simulink subsystem "PID_controller_subsys"  (R2022b)
settings: Solver=VariableStepAuto  StartTime=0.0  StopTime=10.0  RelTol=1e-3
settings Model: Creator=seobokyeong  LastModifiedBy=kevin

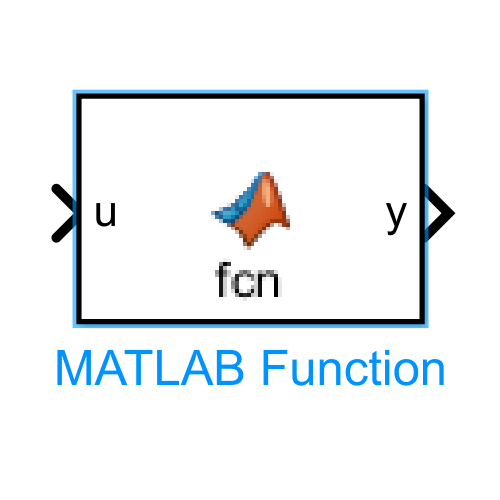
[thumbnail: Simulink's stored preview of the top-level diagram]
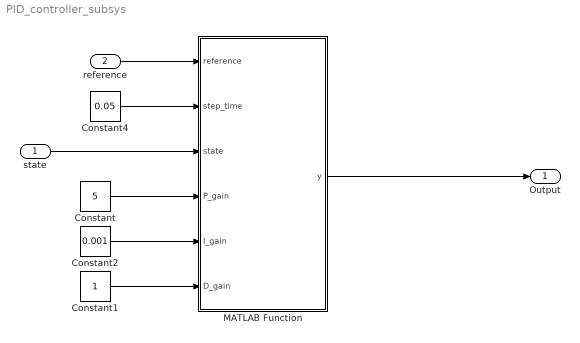
== system PID_controller_subsys ==
  state : Inport
  reference : Inport  Port=2
  Constant : Constant  Value=5
  Constant1 : Constant
  Constant2 : Constant  Value=0.001
  Constant4 : Constant  Value=0.05
  MATLAB Function : MATLAB Function  TreatAsAtomicUnit=on
  Output : Outport
  wires:
  Constant2/1 -> MATLAB Function/5(I_gain)
  Constant1/1 -> MATLAB Function/6(D_gain)
  Constant/1 -> MATLAB Function/4(P_gain)
  MATLAB Function/1(y) -> Output/1
  state/1 -> MATLAB Function/3(state)
  Constant4/1 -> MATLAB Function/2(step_time)
  reference/1 -> MATLAB Function/1(reference)

== matlab function PID_controller_subsys/MATLAB Function ==
  data: reference input; step_time input; y output; state input; P_gain input; I_gain input; D_gain input
function y = PID_controller_subsys(reference, step_time, state, P_gain,I_gain,D_gain) 
    y = PID_controller_fcn(reference, step_time, state, P_gain,I_gain,D_gain);
    if abs(y) > 1 %y값은 tan
        y = 0.05*y/abs(y);
    end

    if abs(y) < 0.01
        y = 0;
    end
end
